simulink model "uz_mlp_three_layer"  (R2021a)
settings: Solver=FixedStepDiscrete  StartTime=0.0  StopTime=5000  RelTol=1e-3
values from neighbouring files (symbols this model uses):
  nn = nn.set_all_parameter(rand_variables)    [mlp2_definition.m]
  nn_data_type_max = 131071    [mlp2_definition.m]
  numInput = 13    [mlp2_definition.m]
  numOut = 4    [mlp2_definition.m]
libraries: hdlsllib x90, simulink x79, el_machinelearning x2
(part 4 of 4)

== stateflow chart uz_mlp_three_layer/reluLayer_4Parallel/StateMachines1/layer_control ==
  settings: executeAtInitialization=1
  state entry_to_entry_state
    layer_rdy=true;
    counter_rest=true; % reset counter for looping through perceptrons of one layer
  state calc_perceptron
    enable_mac=true;
  state idle
    cnt_enable=false;
  state finished2
    layer_finished=false;
  state perceptron_rdy
    cnt_enable=true;
    counter_rest=false;
  state finished
    layer_finished=true;
  state calc_running
    enable_mac=false;
  (default) -> entry_to_entry_state
  finished2 -> entry_to_entry_state
  entry_to_entry_state -> idle : [ext_enable==true]
  idle -> calc_perceptron : [mac_ready==true ]
  calc_perceptron -> calc_running : [mac_ready==false]
  perceptron_rdy -> idle
  finished -> finished2
  calc_running -> perceptron_rdy [order 1] : [mac_ready==true && cnt_finished==false]
  calc_running -> finished [order 2] : [mac_ready==true & cnt_finished==true]
  data: ext_enable input boolean; enable_mac output boolean; mac_ready input boolean; layer_rdy output boolean; cnt_enable output boolean; counter_rest output boolean; cnt_finished input boolean; layer_finished output
